simulink model "Q4"  (R2021b)
settings: Solver=VariableStepAuto  StartTime=0.0  StopTime=25  RelTol=1e-3
settings Model: Creator=DSDLn  LastModifiedBy=DSDLn

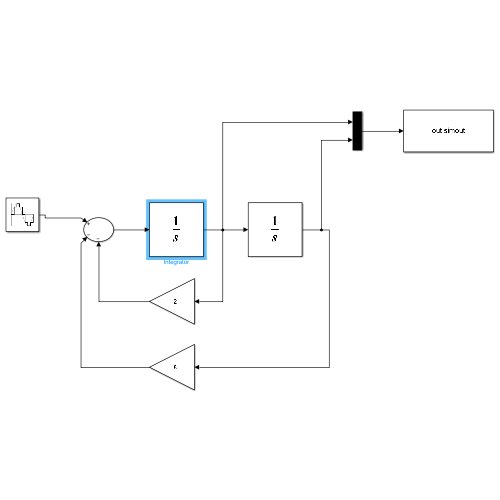
[thumbnail: Simulink's stored preview of the top-level diagram]
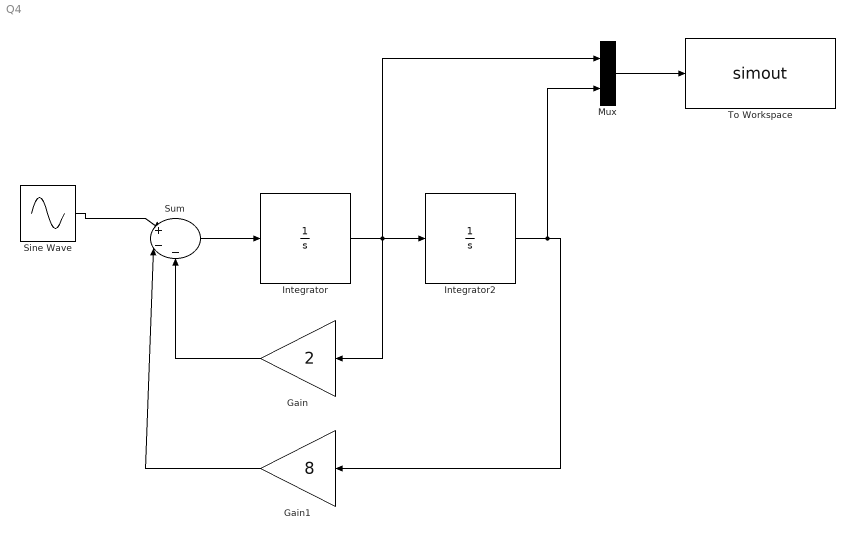
== system Q4 ==
  Gain : Gain  Gain=2
  Gain1 : Gain  Gain=8
  Integrator : Integrator
  Integrator2 : Integrator
  Mux : Mux  Inputs=2
  Sine Wave : Sin  SampleTime=0.01
  Sum : Sum  Inputs=|+--
  To Workspace : ToWorkspace  VariableName=simout  SampleTime=-1
  wires:
  Integrator/1 -> Mux/1, Gain/1, Integrator2/1
  Integrator2/1 -> Mux/2, Gain1/1
  Sum/1 -> Integrator/1
  Gain/1 -> Sum/3
  Gain1/1 -> Sum/2
  Sine Wave/1 -> Sum/1
  Mux/1 -> To Workspace/1
